simulink model "TestesEmSimulink"  (R2018b)
settings: Solver=VariableStepAuto  StartTime=0.0  StopTime=40.0  RelTol=1e-3
values from neighbouring files (symbols this model uses):
  g = (s*eye(size(Apos,1)) - Apos)\(Bpos)    [PontosDeEquilibrioPolimer.m]
libraries: cstblocks x4
settings Model: Creator=lipec  LastModifiedBy=lipec

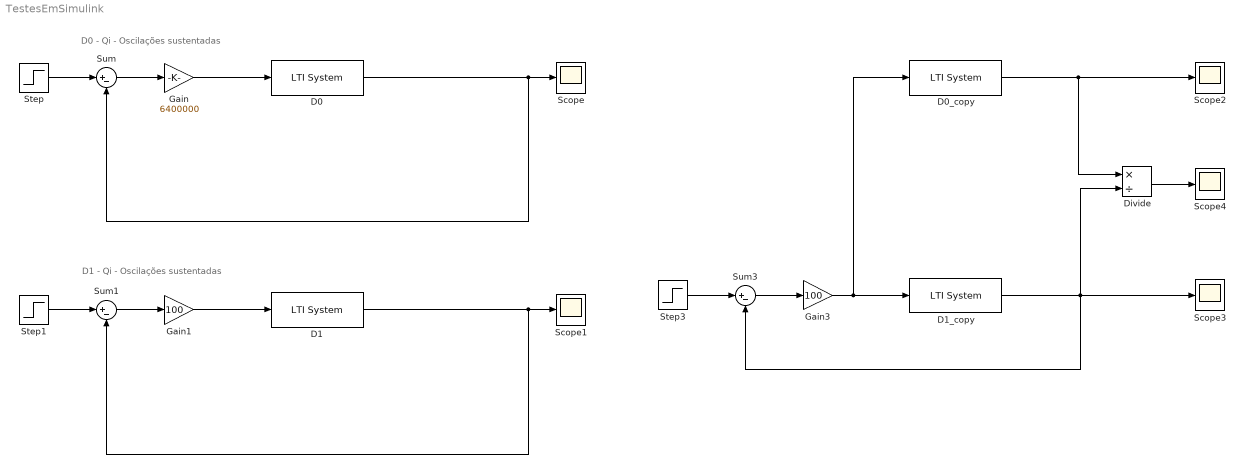
== system TestesEmSimulink ==
  note: D1 - Qi - Oscilações sustentadas
  note: D0 - Qi - Oscilações sustentadas
  D0 : cstblocks/LTI System  sys=g(5,1)  IC=[]
  D0_copy : cstblocks/LTI System  sys=g(5,1)  IC=[]
  D1 : cstblocks/LTI System  sys=g(6,1)  IC=[]
  D1_copy : cstblocks/LTI System  sys=g(6,1)  IC=[]
  Divide : Product  Inputs=*/
  Gain : Gain  Gain=6400000
  Gain1 : Gain  Gain=100
  Gain3 : Gain  Gain=100
  Scope{,1..4} (5 alike) : Scope
  Step : Step  SampleTime=0
  Step1 : Step  SampleTime=0
  Step3 : Step  SampleTime=0
  Sum : Sum  Inputs=|+-
  Sum1 : Sum  Inputs=|+-
  Sum3 : Sum  Inputs=|+-
  wires:
  D0/1 -> Sum/2, Scope/1
  Step/1 -> Sum/1
  Sum/1 -> Gain/1
  Gain/1 -> D0/1
  D1/1 -> Sum1/2, Scope1/1
  Gain1/1 -> D1/1
  Sum1/1 -> Gain1/1
  Step1/1 -> Sum1/1
  D0_copy/1 -> Divide/1, Scope2/1
  Gain3/1 -> D0_copy/1, D1_copy/1
  Step3/1 -> Sum3/1
  Sum3/1 -> Gain3/1
  D1_copy/1 -> Scope3/1, Sum3/2, Divide/2
  Divide/1 -> Scope4/1
